simulink model "magTheta16bit"  (R2020b)
settings: Solver=FixedStepAuto  StartTime=0.0  StopTime=2  RelTol=1e-3
StopFcn:
  | %% Visualize output
  | mag = out.mag.data(:,:,end);
  | theta = out.theta.data(:,:,end);
  | 
  | imwrite(mag,'mag.tif')
  | imwrite(theta,'theta.tif')
values from neighbouring files (symbols this model uses):
  COLS = 752    [setup.m]    (also in setup_old.m = 640)
undefined symbols (not defined in the file or in its folder): gray
libraries: hdlsllib x59, visionhdlio x4, simulink x2, visionsources x1
(part 2 of 2)

== system magTheta16bit/MagTheta/GaussianFilter/Symmetric Filter/Verticle Filter/Symmetry ==
  data_in : Inport
  Add : Sum  Inputs=|++  AccumDataTypeStr=cap_2  OutDataTypeStr=cap_2  RndMeth=Nearest
  Data Type Duplicate : DataTypeDuplicate
  Data Type Conversion : DataTypeConversion
  Demux : Demux  Outputs=3
  Mux : Mux  Inputs=2
  data_out : Outport
  wires:
  Add/1 -> Data Type Duplicate/1, Mux/1
  data_in/1 -> Demux/1
  Demux/3 -> Add/2
  Demux/1 -> Add/1
  Mux/1 -> data_out/1
  Demux/2 -> Data Type Conversion/1
  Data Type Conversion/1 -> Data Type Duplicate/2, Mux/2

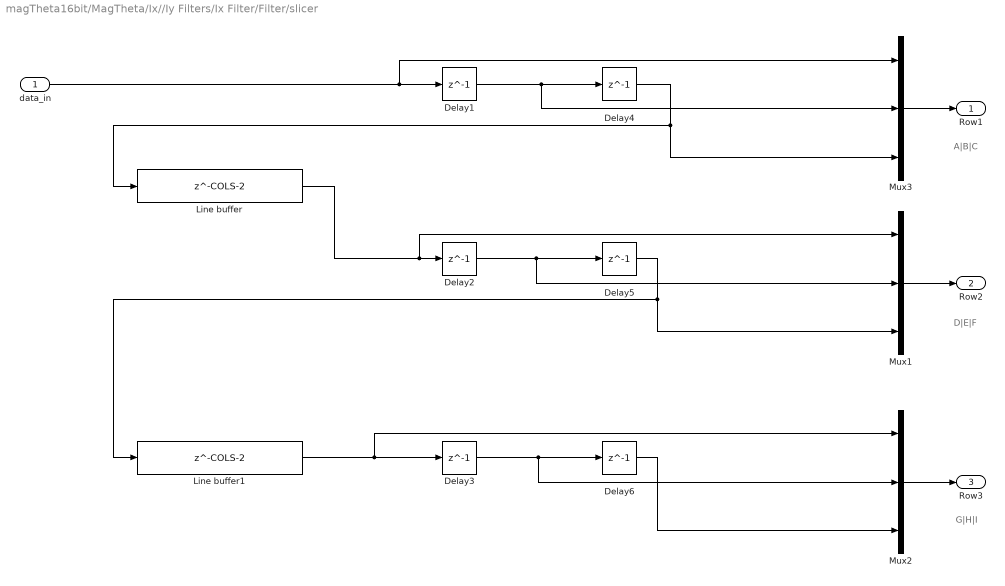
== system magTheta16bit/MagTheta/Ix//Iy Filters/Ix Filter/Filter/slicer ==
  note: A|B|C
  note: D|E|F
  note: G|H|I
  data_in : Inport
  Delay{1..6} (6 alike) : Delay  DelayLength=1  InitialCondition=0
  Line buffer : Delay  DelayLength=COLS-2  InitialCondition=0
  Line buffer1 : Delay  DelayLength=COLS-2  InitialCondition=0
  Mux1 : Mux  Inputs=3
  Mux2 : Mux  Inputs=3
  Mux3 : Mux  Inputs=3
  Row1 : Outport  VectorParamsAs1DForOutWhenUnconnected=off
  Row2 : Outport  Port=2  VectorParamsAs1DForOutWhenUnconnected=off
  Row3 : Outport  Port=3  VectorParamsAs1DForOutWhenUnconnected=off
  wires:
  Delay4/1 -> Mux3/3, Line buffer/1
  data_in/1 -> Mux3/1, Delay1/1
  Delay1/1 -> Mux3/2, Delay4/1
  Delay3/1 -> Mux2/2, Delay6/1
  Delay5/1 -> Mux1/3, Line buffer1/1
  Delay6/1 -> Mux2/3
  Line buffer/1 -> Mux1/1, Delay2/1
  Line buffer1/1 -> Mux2/1, Delay3/1
  Delay2/1 -> Mux1/2, Delay5/1
  Mux1/1 -> Row2/1
  Mux2/1 -> Row3/1
  Mux3/1 -> Row1/1

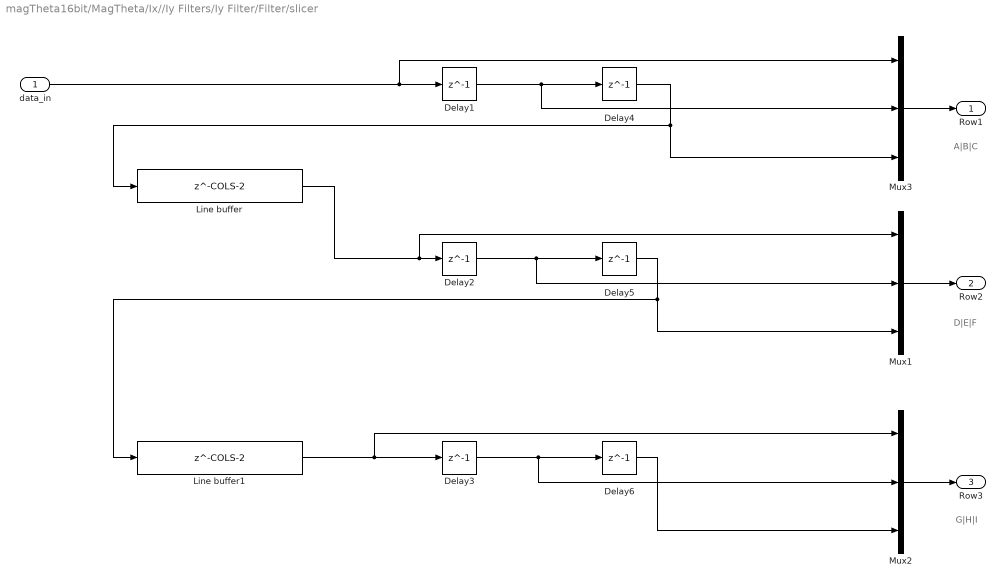
== system magTheta16bit/MagTheta/Ix//Iy Filters/Iy Filter/Filter/slicer ==
  note: A|B|C
  note: D|E|F
  note: G|H|I
  data_in : Inport
  Delay{1..6} (6 alike) : Delay  DelayLength=1  InitialCondition=0
  Line buffer : Delay  DelayLength=COLS-2  InitialCondition=0
  Line buffer1 : Delay  DelayLength=COLS-2  InitialCondition=0
  Mux1 : Mux  Inputs=3
  Mux2 : Mux  Inputs=3
  Mux3 : Mux  Inputs=3
  Row1 : Outport  VectorParamsAs1DForOutWhenUnconnected=off
  Row2 : Outport  Port=2  VectorParamsAs1DForOutWhenUnconnected=off
  Row3 : Outport  Port=3  VectorParamsAs1DForOutWhenUnconnected=off
  wires:
  Delay4/1 -> Mux3/3, Line buffer/1
  data_in/1 -> Mux3/1, Delay1/1
  Delay1/1 -> Mux3/2, Delay4/1
  Delay3/1 -> Mux2/2, Delay6/1
  Delay5/1 -> Mux1/3, Line buffer1/1
  Delay6/1 -> Mux2/3
  Line buffer/1 -> Mux1/1, Delay2/1
  Line buffer1/1 -> Mux2/1, Delay3/1
  Delay2/1 -> Mux1/2, Delay5/1
  Mux1/1 -> Row2/1
  Mux2/1 -> Row3/1
  Mux3/1 -> Row1/1
